simulink model "dds_cwg_32k_nb_half"  (R2018a)
settings: Solver=VariableStepDiscrete  StartTime=0.0  StopTime=(2^16)*20  RelTol=1e-3
undefined symbols (not defined in the file or in its folder): fft_stages, pfb_coeff_gen_calc
libraries: xbsIndex_r4 x11238, casper_library_misc x13, casper_library_delays x2, xps_library x1
(part 14 of 69)

== system dds_cwg_32k_nb_half/DDC/dec_fir_async1 ==
  sync_in : Inport
  dv_in : Inport  Port=2
  real1 : Inport  Port=3
  imag1 : Inport  Port=4
  real2 : Inport  Port=5
  imag2 : Inport  Port=6
  real3 : Inport  Port=7
  imag3 : Inport  Port=8
  real4 : Inport  Port=9
  imag4 : Inport  Port=10
  real5 : Inport  Port=11
  imag5 : Inport  Port=12
  real6 : Inport  Port=13
  imag6 : Inport  Port=14
  real7 : Inport  Port=15
  imag7 : Inport  Port=16
  real8 : Inport  Port=17
  imag8 : Inport  Port=18
  real9 : Inport  Port=19
  imag9 : Inport  Port=20
  real10 : Inport  Port=21
  imag10 : Inport  Port=22
  real11 : Inport  Port=23
  imag11 : Inport  Port=24
  real12 : Inport  Port=25
  imag12 : Inport  Port=26
  real13 : Inport  Port=27
  imag13 : Inport  Port=28
  real14 : Inport  Port=29
  imag14 : Inport  Port=30
  real15 : Inport  Port=31
  imag15 : Inport  Port=32
  real16 : Inport  Port=33
  imag16 : Inport  Port=34
  real17 : Inport  Port=35
  imag17 : Inport  Port=36
  real18 : Inport  Port=37
  imag18 : Inport  Port=38
  real19 : Inport  Port=39
  imag19 : Inport  Port=40
  real20 : Inport  Port=41
  imag20 : Inport  Port=42
  real21 : Inport  Port=43
  imag21 : Inport  Port=44
  real22 : Inport  Port=45
  imag22 : Inport  Port=46
  real23 : Inport  Port=47
  imag23 : Inport  Port=48
  real24 : Inport  Port=49
  imag24 : Inport  Port=50
  real25 : Inport  Port=51
  imag25 : Inport  Port=52
  real26 : Inport  Port=53
  imag26 : Inport  Port=54
  real27 : Inport  Port=55
  imag27 : Inport  Port=56
  real28 : Inport  Port=57
  imag28 : Inport  Port=58
  real29 : Inport  Port=59
  imag29 : Inport  Port=60
  real30 : Inport  Port=61
  imag30 : Inport  Port=62
  real31 : Inport  Port=63
  imag31 : Inport  Port=64
  real32 : Inport  Port=65
  imag32 : Inport  Port=66
  convert1 : xbsIndex_r4/Convert  gui_display_data_type=Fixed-point  arith_type="Signed  (2's comp)"  n_bits=18  bin_pt=17  float_type=Single  exp_bits=8  fraction_bits=24  quantization="Round  (unbiased: +/- Inf)"  overflow=Wrap  en=off  latency=7  pipeline=off  dbl_ovrd=off  block_type=convert
  convert2 : xbsIndex_r4/Convert  gui_display_data_type=Fixed-point  arith_type="Signed  (2's comp)"  n_bits=18  bin_pt=17  float_type=Single  exp_bits=8  fraction_bits=24  quantization="Round  (unbiased: +/- Inf)"  overflow=Wrap  en=off  latency=7  pipeline=off  dbl_ovrd=off  block_type=convert
  dv_delay : xbsIndex_r4/Delay  rst=off  infoeditControl=Selection of Reset will increase slice count due to use of real FFs and instead of SRLs  en=off  latency=2  reg_retiming=off  dbl_ovrd=off  block_type=delay
  fir_col_async1 : Subsystem  AncestorBlock=casper_library_downconverter/fir_col_async  mask(fir_col_async){n_inputs=32, coeff=[-0.001506    -0.00204   -0.002487    -0.00285   -0.003135   -0.003345   -0.003487   -0.003566   -0.003589   -0.003562   -0.003491   -0.003383   -0.003243   -0.003077   -0.002892   -0.002692   -0.002483   -0.002269   -0.002054   -0.001841   -0.001634   -0.001436   -0.001247   -0.001071   -0.000909    -0.00076   -0.000626   -0.000507   -0.000402   -0.000312   -0.000234   -0.000339], add_latency=7, mult_latency=7, coeff_bit_width=18, coeff_bin_pt=17, first_stage_hdl=on, adder_imp=DSP48, async=on, bus_input=off, input_width=0, input_bp=0, input_type=Signed, dbl=on}
      mask prompts: n_inputs "Inputs"; coeff "Coefficients"; add_latency "Add latency"; mult_latency "Mult Latency"; coeff_bit_width "Coefficient bit width"; coeff_bin_pt "Coefficient binary point"; first_stage_hdl "Implement first stage of adder trees on output as behavioural HDL"; adder_imp "Adder implementation"; async "Asynchronous ops"; bus_input "Bus input"; input_width "Input bitwidth"; input_bp "Input binary point"; input_type "Input datatype"; dbl "Double col"
      mask init:
      | fir_col_async_init(gcb);
      mask Help: eval('xlWeb(''http://casper.berkeley.edu/wiki/Fir_col'')')
      mask TypeOptions adder_imp: Behavioral | Fabric | DSP48
      mask Callback bus_input:
      | onoff = get_param(gcb, 'bus_input');
      | set_param_state(gcb, 'input_width', onoff)
      | set_param_state(gcb, 'input_bp', onoff)
      | set_param_state(gcb, 'input_type', onoff)
      mask TypeOptions input_type: Signed | Unsigned
  fir_col_async2 : Subsystem  AncestorBlock=casper_library_downconverter/fir_col_async  mask(fir_col_async){n_inputs=32, coeff=[0.035749    0.035589    0.035272    0.034799    0.034177     0.03341    0.032507    0.031476    0.030327    0.029072     0.02772    0.026286    0.024783    0.023223     0.02162    0.019988    0.018341    0.016693    0.015055     0.01344     0.01186    0.010325    0.008847    0.007432    0.006089    0.004826    0.003646    0.002555    0.001555    0.000649   -0.000163   -0.000881], add_latency=7, mult_latency=7, coeff_bit_width=18, coeff_bin_pt=17, first_stage_hdl=on, adder_imp=DSP48, async=on, bus_input=off, input_width=0, input_bp=0, input_type=Signed, dbl=on}
      mask prompts: n_inputs "Inputs"; coeff "Coefficients"; add_latency "Add latency"; mult_latency "Mult Latency"; coeff_bit_width "Coefficient bit width"; coeff_bin_pt "Coefficient binary point"; first_stage_hdl "Implement first stage of adder trees on output as behavioural HDL"; adder_imp "Adder implementation"; async "Asynchronous ops"; bus_input "Bus input"; input_width "Input bitwidth"; input_bp "Input binary point"; input_type "Input datatype"; dbl "Double col"
      mask init:
      | fir_col_async_init(gcb);
      mask Help: eval('xlWeb(''http://casper.berkeley.edu/wiki/Fir_col'')')
      mask TypeOptions adder_imp: Behavioral | Fabric | DSP48
      mask Callback bus_input:
      | onoff = get_param(gcb, 'bus_input');
      | set_param_state(gcb, 'input_width', onoff)
      | set_param_state(gcb, 'input_bp', onoff)
      | set_param_state(gcb, 'input_type', onoff)
      mask TypeOptions input_type: Signed | Unsigned
  imag_sum : Subsystem  AncestorBlock=casper_library_misc/adder_tree  mask(adder_tree){n_inputs=2, csp_latency=7, adder_imp=DSP48, first_stage_hdl=off, floating_point=off, dvalid_en=on, float_type=single, frac_width=0, exp_width=0}
      mask prompts: n_inputs "Number of Inputs"; csp_latency "Add Latency"; adder_imp "Adder implementation"; first_stage_hdl "Use behavioural HDL for first stage of adders"; floating_point "floating point"; float_type "float type"; frac_width "fraction length"; exp_width "exponent length"
      mask help:
      | Sums all inputs using a tree of adds and delays.
      |
      | Number of inputs: The number of inputs to the block to be summed
      | Add latency: The number of clock cycles to perform one addition (affects timing)..
      | Adder implementation: choice of fabric or DSP48E core, or behavioral HDL
      | Use behavioural HDL for first stage of adders: Causes the first stage of adders to be absorbed into DSP blocks if multipliers precede them (Virtex 5). Overrides Adder implementation
      mask init:
      | adder_tree_init(gcb, ...
      |     'n_inputs', n_inputs, ...
      |     'csp_latency', csp_latency, ...
      |     'adder_imp', adder_imp, ...
      |     'dvalid_en', dvalid_en, ...
      |     'floating_point', floating_point, ...
      |     'float_type', float_type, ...
      |     'exp_width', exp_width, ...
      |     'frac_width', frac_width, ...     
      |     'first_stage_hdl', first_stage_hdl);
      settings: AttributesFormatString=latency 7
      mask Help: eval('xlWeb(''http://casper.berkeley.edu/wiki/Adder_tree'')')
      mask TypeOptions adder_imp: Behavioral | Fabric | DSP48
      mask Callback floating_point:
      | onoff = get_param(gcb, 'floating_point');
      | if strcmp(onoff,'on')
      |     enable_fixpt = 'off'
      |     set_param_state(gcb, 'float_type', 'on')
      | 
      |     f_type = get_param(gcb, 'float_type')
      |     if strcmp(f_type,'custom')
      |         set_param_state(gcb, 'exp_width', 'on')
      |         set_param_state(gcb, 'frac_width', 'on')
      |     else
      |         set_param_state(gcb, 'exp_width', 'off')
      |         set_param_state(gcb, 'frac_width', 'off')
      |     end
      | 
      | 
      | else
      |     enable_fixpt = 'on'
      |     set_param_state(gcb, 'float_type', 'off')
      |     set_param_state(gcb, 'exp_width', 'off')
      |     set_param_state(gcb, 'frac_width', 'off')
      | end
      mask TypeOptions float_type: single | custom
      mask Callback float_type:
      | f_type = get_param(gcb, 'float_type')
      | if strcmp(f_type,'custom')
      |     set_param_state(gcb, 'exp_width', 'on')
      |     set_param_state(gcb, 'frac_width', 'on')
      | else
      |     set_param_state(gcb, 'exp_width', 'off')
      |     set_param_state(gcb, 'frac_width', 'off')
      | end
  real_sum : Subsystem  AncestorBlock=casper_library_misc/adder_tree  mask(adder_tree){n_inputs=2, csp_latency=7, adder_imp=DSP48, first_stage_hdl=off, floating_point=off, dvalid_en=on, float_type=single, frac_width=0, exp_width=0}
      mask prompts: n_inputs "Number of Inputs"; csp_latency "Add Latency"; adder_imp "Adder implementation"; first_stage_hdl "Use behavioural HDL for first stage of adders"; floating_point "floating point"; float_type "float type"; frac_width "fraction length"; exp_width "exponent length"
      mask help:
      | Sums all inputs using a tree of adds and delays.
      |
      | Number of inputs: The number of inputs to the block to be summed
      | Add latency: The number of clock cycles to perform one addition (affects timing)..
      | Adder implementation: choice of fabric or DSP48E core, or behavioral HDL
      | Use behavioural HDL for first stage of adders: Causes the first stage of adders to be absorbed into DSP blocks if multipliers precede them (Virtex 5). Overrides Adder implementation
      mask init: same as dds_cwg_32k_nb_half/DDC/dec_fir_async1/imag_sum
      settings: AttributesFormatString=latency 7
      mask Help: eval('xlWeb(''http://casper.berkeley.edu/wiki/Adder_tree'')')
      mask TypeOptions adder_imp: Behavioral | Fabric | DSP48
      mask Callback floating_point:
      | onoff = get_param(gcb, 'floating_point');
      | if strcmp(onoff,'on')
      |     enable_fixpt = 'off'
      |     set_param_state(gcb, 'float_type', 'on')
      | 
      |     f_type = get_param(gcb, 'float_type')
      |     if strcmp(f_type,'custom')
      |         set_param_state(gcb, 'exp_width', 'on')
      |         set_param_state(gcb, 'frac_width', 'on')
      |     else
      |         set_param_state(gcb, 'exp_width', 'off')
      |         set_param_state(gcb, 'frac_width', 'off')
      |     end
      | 
      | 
      | else
      |     enable_fixpt = 'on'
      |     set_param_state(gcb, 'float_type', 'off')
      |     set_param_state(gcb, 'exp_width', 'off')
      |     set_param_state(gcb, 'frac_width', 'off')
      | end
      mask TypeOptions float_type: single | custom
      mask Callback float_type:
      | f_type = get_param(gcb, 'float_type')
      | if strcmp(f_type,'custom')
      |     set_param_state(gcb, 'exp_width', 'on')
      |     set_param_state(gcb, 'frac_width', 'on')
      | else
      |     set_param_state(gcb, 'exp_width', 'off')
      |     set_param_state(gcb, 'frac_width', 'off')
      | end
  ri_to_c : casper_library_misc/ri_to_c
      settings: SourceProductName=CASPER DSP Blockset
  shift1 : xbsIndex_r4/Shift  shift_dir=Left  shift_bits=1  en=off  latency=1  precision=Full  arith_type="Signed  (2's comp)"  n_bits=16  bin_pt=14  quantization=Truncate  overflow=Wrap  dbl_ovrd=off  block_type=shift
  shift2 : xbsIndex_r4/Shift  shift_dir=Left  shift_bits=1  en=off  latency=1  precision=Full  arith_type="Signed  (2's comp)"  n_bits=16  bin_pt=14  quantization=Truncate  overflow=Wrap  dbl_ovrd=off  block_type=shift
  sync_delay : xbsIndex_r4/Delay  rst=off  infoeditControl=Selection of Reset will increase slice count due to use of real FFs and instead of SRLs  en=on  latency=56  reg_retiming=off  dbl_ovrd=off  block_type=delay
  sync_out : Outport
  dout : Outport  Port=2
  dv_out : Outport  Port=3
  wires:
  sync_in/1 -> sync_delay/1
  dv_in/1 -> dv_delay/1, sync_delay/2, fir_col_async1/129(dv), fir_col_async2/129(dv), real_sum/1(dv_in), imag_sum/1(dv_in)
  dv_delay/1 -> dv_out/1
  real1/1 -> fir_col_async1/1(real1)
  imag1/1 -> fir_col_async1/2(imag1)
  real2/1 -> fir_col_async1/3(real2)
  imag2/1 -> fir_col_async1/4(imag2)
  real3/1 -> fir_col_async1/5(real3)
  imag3/1 -> fir_col_async1/6(imag3)
  real4/1 -> fir_col_async1/7(real4)
  imag4/1 -> fir_col_async1/8(imag4)
  real5/1 -> fir_col_async1/9(real5)
  imag5/1 -> fir_col_async1/10(imag5)
  real6/1 -> fir_col_async1/11(real6)
  imag6/1 -> fir_col_async1/12(imag6)
  real7/1 -> fir_col_async1/13(real7)
  imag7/1 -> fir_col_async1/14(imag7)
  real8/1 -> fir_col_async1/15(real8)
  imag8/1 -> fir_col_async1/16(imag8)
  real9/1 -> fir_col_async1/17(real9)
  imag9/1 -> fir_col_async1/18(imag9)
  real10/1 -> fir_col_async1/19(real10)
  imag10/1 -> fir_col_async1/20(imag10)
  real11/1 -> fir_col_async1/21(real11)
  imag11/1 -> fir_col_async1/22(imag11)
  real12/1 -> fir_col_async1/23(real12)
  imag12/1 -> fir_col_async1/24(imag12)
  real13/1 -> fir_col_async1/25(real13)
  imag13/1 -> fir_col_async1/26(imag13)
  real14/1 -> fir_col_async1/27(real14)
  imag14/1 -> fir_col_async1/28(imag14)
  real15/1 -> fir_col_async1/29(real15)
  imag15/1 -> fir_col_async1/30(imag15)
  real16/1 -> fir_col_async1/31(real16)
  imag16/1 -> fir_col_async1/32(imag16)
  real17/1 -> fir_col_async1/33(real17)
  imag17/1 -> fir_col_async1/34(imag17)
  real18/1 -> fir_col_async1/35(real18)
  imag18/1 -> fir_col_async1/36(imag18)
  real19/1 -> fir_col_async1/37(real19)
  imag19/1 -> fir_col_async1/38(imag19)
  real20/1 -> fir_col_async1/39(real20)
  imag20/1 -> fir_col_async1/40(imag20)
  real21/1 -> fir_col_async1/41(real21)
  imag21/1 -> fir_col_async1/42(imag21)
  real22/1 -> fir_col_async1/43(real22)
  imag22/1 -> fir_col_async1/44(imag22)
  real23/1 -> fir_col_async1/45(real23)
  imag23/1 -> fir_col_async1/46(imag23)
  real24/1 -> fir_col_async1/47(real24)
  imag24/1 -> fir_col_async1/48(imag24)
  real25/1 -> fir_col_async1/49(real25)
  imag25/1 -> fir_col_async1/50(imag25)
  real26/1 -> fir_col_async1/51(real26)
  imag26/1 -> fir_col_async1/52(imag26)
  real27/1 -> fir_col_async1/53(real27)
  imag27/1 -> fir_col_async1/54(imag27)
  real28/1 -> fir_col_async1/55(real28)
  imag28/1 -> fir_col_async1/56(imag28)
  real29/1 -> fir_col_async1/57(real29)
  imag29/1 -> fir_col_async1/58(imag29)
  real30/1 -> fir_col_async1/59(real30)
  imag30/1 -> fir_col_async1/60(imag30)
  real31/1 -> fir_col_async1/61(real31)
  imag31/1 -> fir_col_async1/62(imag31)
  real32/1 -> fir_col_async1/63(real32)
  imag32/1 -> fir_col_async1/64(imag32)
  fir_col_async1/129(real_sum) -> real_sum/3(din1)
  fir_col_async1/130(imag_sum) -> imag_sum/3(din1)
  fir_col_async1/1(real_out1) -> fir_col_async2/1(real1)
  fir_col_async1/2(imag_out1) -> fir_col_async2/2(imag1)
  fir_col_async1/3(real_out2) -> fir_col_async2/3(real2)
  fir_col_async1/4(imag_out2) -> fir_col_async2/4(imag2)
  fir_col_async1/5(real_out3) -> fir_col_async2/5(real3)
  fir_col_async1/6(imag_out3) -> fir_col_async2/6(imag3)
  fir_col_async1/7(real_out4) -> fir_col_async2/7(real4)
  fir_col_async1/8(imag_out4) -> fir_col_async2/8(imag4)
  fir_col_async1/9(real_out5) -> fir_col_async2/9(real5)
  fir_col_async1/10(imag_out5) -> fir_col_async2/10(imag5)
  fir_col_async1/11(real_out6) -> fir_col_async2/11(real6)
  fir_col_async1/12(imag_out6) -> fir_col_async2/12(imag6)
  fir_col_async1/13(real_out7) -> fir_col_async2/13(real7)
  fir_col_async1/14(imag_out7) -> fir_col_async2/14(imag7)
  fir_col_async1/15(real_out8) -> fir_col_async2/15(real8)
  fir_col_async1/16(imag_out8) -> fir_col_async2/16(imag8)
  fir_col_async1/17(real_out9) -> fir_col_async2/17(real9)
  fir_col_async1/18(imag_out9) -> fir_col_async2/18(imag9)
  fir_col_async1/19(real_out10) -> fir_col_async2/19(real10)
  fir_col_async1/20(imag_out10) -> fir_col_async2/20(imag10)
  fir_col_async1/21(real_out11) -> fir_col_async2/21(real11)
  fir_col_async1/22(imag_out11) -> fir_col_async2/22(imag11)
  fir_col_async1/23(real_out12) -> fir_col_async2/23(real12)
  fir_col_async1/24(imag_out12) -> fir_col_async2/24(imag12)
  fir_col_async1/25(real_out13) -> fir_col_async2/25(real13)
  fir_col_async1/26(imag_out13) -> fir_col_async2/26(imag13)
  fir_col_async1/27(real_out14) -> fir_col_async2/27(real14)
  fir_col_async1/28(imag_out14) -> fir_col_async2/28(imag14)
  fir_col_async1/29(real_out15) -> fir_col_async2/29(real15)
  fir_col_async1/30(imag_out15) -> fir_col_async2/30(imag15)
  fir_col_async1/31(real_out16) -> fir_col_async2/31(real16)
  fir_col_async1/32(imag_out16) -> fir_col_async2/32(imag16)
  fir_col_async1/33(real_out17) -> fir_col_async2/33(real17)
  fir_col_async1/34(imag_out17) -> fir_col_async2/34(imag17)
  fir_col_async1/35(real_out18) -> fir_col_async2/35(real18)
  fir_col_async1/36(imag_out18) -> fir_col_async2/36(imag18)
  fir_col_async1/37(real_out19) -> fir_col_async2/37(real19)
  fir_col_async1/38(imag_out19) -> fir_col_async2/38(imag19)
  fir_col_async1/39(real_out20) -> fir_col_async2/39(real20)
  fir_col_async1/40(imag_out20) -> fir_col_async2/40(imag20)
  fir_col_async1/41(real_out21) -> fir_col_async2/41(real21)
  fir_col_async1/42(imag_out21) -> fir_col_async2/42(imag21)
  fir_col_async1/43(real_out22) -> fir_col_async2/43(real22)
  fir_col_async1/44(imag_out22) -> fir_col_async2/44(imag22)
  fir_col_async1/45(real_out23) -> fir_col_async2/45(real23)
  fir_col_async1/46(imag_out23) -> fir_col_async2/46(imag23)
  fir_col_async1/47(real_out24) -> fir_col_async2/47(real24)
  fir_col_async1/48(imag_out24) -> fir_col_async2/48(imag24)
  fir_col_async1/49(real_out25) -> fir_col_async2/49(real25)
  fir_col_async1/50(imag_out25) -> fir_col_async2/50(imag25)
  fir_col_async1/51(real_out26) -> fir_col_async2/51(real26)
  fir_col_async1/52(imag_out26) -> fir_col_async2/52(imag26)
  fir_col_async1/53(real_out27) -> fir_col_async2/53(real27)
  fir_col_async1/54(imag_out27) -> fir_col_async2/54(imag27)
  fir_col_async1/55(real_out28) -> fir_col_async2/55(real28)
  fir_col_async1/56(imag_out28) -> fir_col_async2/56(imag28)
  fir_col_async1/57(real_out29) -> fir_col_async2/57(real29)
  fir_col_async1/58(imag_out29) -> fir_col_async2/58(imag29)
  fir_col_async1/59(real_out30) -> fir_col_async2/59(real30)
  fir_col_async1/60(imag_out30) -> fir_col_async2/60(imag30)
  fir_col_async1/61(real_out31) -> fir_col_async2/61(real31)
  fir_col_async1/62(imag_out31) -> fir_col_async2/62(imag31)
  fir_col_async1/63(real_out32) -> fir_col_async2/63(real32)
  fir_col_async1/64(imag_out32) -> fir_col_async2/64(imag32)
  fir_col_async2/129(real_sum) -> real_sum/4(din2)
  fir_col_async2/130(imag_sum) -> imag_sum/4(din2)
  real_sum/2(dout) -> shift1/1
  imag_sum/2(dout) -> shift2/1
  shift1/1 -> convert1/1
  shift2/1 -> convert2/1
  convert1/1 -> ri_to_c/1
  convert2/1 -> ri_to_c/2
  ri_to_c/1 -> dout/1
  real_sum/1(sync_out) -> sync_out/1
  sync_delay/1 -> real_sum/2(sync), imag_sum/2(sync)
  fir_col_async2/65(real_back_out1) -> fir_col_async1/65(real_back1)
  fir_col_async2/66(imag_back_out1) -> fir_col_async1/66(imag_back1)
  fir_col_async2/67(real_back_out2) -> fir_col_async1/67(real_back2)
  fir_col_async2/68(imag_back_out2) -> fir_col_async1/68(imag_back2)
  fir_col_async2/69(real_back_out3) -> fir_col_async1/69(real_back3)
  fir_col_async2/70(imag_back_out3) -> fir_col_async1/70(imag_back3)
  fir_col_async2/71(real_back_out4) -> fir_col_async1/71(real_back4)
  fir_col_async2/72(imag_back_out4) -> fir_col_async1/72(imag_back4)
  fir_col_async2/73(real_back_out5) -> fir_col_async1/73(real_back5)
  fir_col_async2/74(imag_back_out5) -> fir_col_async1/74(imag_back5)
  fir_col_async2/75(real_back_out6) -> fir_col_async1/75(real_back6)
  fir_col_async2/76(imag_back_out6) -> fir_col_async1/76(imag_back6)
  fir_col_async2/77(real_back_out7) -> fir_col_async1/77(real_back7)
  fir_col_async2/78(imag_back_out7) -> fir_col_async1/78(imag_back7)
  fir_col_async2/79(real_back_out8) -> fir_col_async1/79(real_back8)
  fir_col_async2/80(imag_back_out8) -> fir_col_async1/80(imag_back8)
  fir_col_async2/81(real_back_out9) -> fir_col_async1/81(real_back9)
  fir_col_async2/82(imag_back_out9) -> fir_col_async1/82(imag_back9)
  fir_col_async2/83(real_back_out10) -> fir_col_async1/83(real_back10)
  fir_col_async2/84(imag_back_out10) -> fir_col_async1/84(imag_back10)
  fir_col_async2/85(real_back_out11) -> fir_col_async1/85(real_back11)
  fir_col_async2/86(imag_back_out11) -> fir_col_async1/86(imag_back11)
  fir_col_async2/87(real_back_out12) -> fir_col_async1/87(real_back12)
  fir_col_async2/88(imag_back_out12) -> fir_col_async1/88(imag_back12)
  fir_col_async2/89(real_back_out13) -> fir_col_async1/89(real_back13)
  fir_col_async2/90(imag_back_out13) -> fir_col_async1/90(imag_back13)
  fir_col_async2/91(real_back_out14) -> fir_col_async1/91(real_back14)
  fir_col_async2/92(imag_back_out14) -> fir_col_async1/92(imag_back14)
  fir_col_async2/93(real_back_out15) -> fir_col_async1/93(real_back15)
  fir_col_async2/94(imag_back_out15) -> fir_col_async1/94(imag_back15)
  fir_col_async2/95(real_back_out16) -> fir_col_async1/95(real_back16)
  fir_col_async2/96(imag_back_out16) -> fir_col_async1/96(imag_back16)
  fir_col_async2/97(real_back_out17) -> fir_col_async1/97(real_back17)
  fir_col_async2/98(imag_back_out17) -> fir_col_async1/98(imag_back17)
  fir_col_async2/99(real_back_out18) -> fir_col_async1/99(real_back18)
  fir_col_async2/100(imag_back_out18) -> fir_col_async1/100(imag_back18)
  fir_col_async2/101(real_back_out19) -> fir_col_async1/101(real_back19)
  fir_col_async2/102(imag_back_out19) -> fir_col_async1/102(imag_back19)
  fir_col_async2/103(real_back_out20) -> fir_col_async1/103(real_back20)
  fir_col_async2/104(imag_back_out20) -> fir_col_async1/104(imag_back20)
  fir_col_async2/105(real_back_out21) -> fir_col_async1/105(real_back21)
  fir_col_async2/106(imag_back_out21) -> fir_col_async1/106(imag_back21)
  fir_col_async2/107(real_back_out22) -> fir_col_async1/107(real_back22)
  fir_col_async2/108(imag_back_out22) -> fir_col_async1/108(imag_back22)
  fir_col_async2/109(real_back_out23) -> fir_col_async1/109(real_back23)
  fir_col_async2/110(imag_back_out23) -> fir_col_async1/110(imag_back23)
  fir_col_async2/111(real_back_out24) -> fir_col_async1/111(real_back24)
  fir_col_async2/112(imag_back_out24) -> fir_col_async1/112(imag_back24)
  fir_col_async2/113(real_back_out25) -> fir_col_async1/113(real_back25)
  fir_col_async2/114(imag_back_out25) -> fir_col_async1/114(imag_back25)
  fir_col_async2/115(real_back_out26) -> fir_col_async1/115(real_back26)
  fir_col_async2/116(imag_back_out26) -> fir_col_async1/116(imag_back26)
  fir_col_async2/117(real_back_out27) -> fir_col_async1/117(real_back27)
  fir_col_async2/118(imag_back_out27) -> fir_col_async1/118(imag_back27)
  fir_col_async2/119(real_back_out28) -> fir_col_async1/119(real_back28)
  fir_col_async2/120(imag_back_out28) -> fir_col_async1/120(imag_back28)
  fir_col_async2/121(real_back_out29) -> fir_col_async1/121(real_back29)
  fir_col_async2/122(imag_back_out29) -> fir_col_async1/122(imag_back29)
  fir_col_async2/123(real_back_out30) -> fir_col_async1/123(real_back30)
  fir_col_async2/124(imag_back_out30) -> fir_col_async1/124(imag_back30)
  fir_col_async2/125(real_back_out31) -> fir_col_async1/125(real_back31)
  fir_col_async2/126(imag_back_out31) -> fir_col_async1/126(imag_back31)
  fir_col_async2/127(real_back_out32) -> fir_col_async1/127(real_back32)
  fir_col_async2/128(imag_back_out32) -> fir_col_async1/128(imag_back32)
  fir_col_async2/1(real_out1) -> fir_col_async2/65(real_back1)
  fir_col_async2/2(imag_out1) -> fir_col_async2/66(imag_back1)
  fir_col_async2/3(real_out2) -> fir_col_async2/67(real_back2)
  fir_col_async2/4(imag_out2) -> fir_col_async2/68(imag_back2)
  fir_col_async2/5(real_out3) -> fir_col_async2/69(real_back3)
  fir_col_async2/6(imag_out3) -> fir_col_async2/70(imag_back3)
  fir_col_async2/7(real_out4) -> fir_col_async2/71(real_back4)
  fir_col_async2/8(imag_out4) -> fir_col_async2/72(imag_back4)
  fir_col_async2/9(real_out5) -> fir_col_async2/73(real_back5)
  fir_col_async2/10(imag_out5) -> fir_col_async2/74(imag_back5)
  fir_col_async2/11(real_out6) -> fir_col_async2/75(real_back6)
  fir_col_async2/12(imag_out6) -> fir_col_async2/76(imag_back6)
  fir_col_async2/13(real_out7) -> fir_col_async2/77(real_back7)
  fir_col_async2/14(imag_out7) -> fir_col_async2/78(imag_back7)
  fir_col_async2/15(real_out8) -> fir_col_async2/79(real_back8)
  fir_col_async2/16(imag_out8) -> fir_col_async2/80(imag_back8)
  fir_col_async2/17(real_out9) -> fir_col_async2/81(real_back9)
  fir_col_async2/18(imag_out9) -> fir_col_async2/82(imag_back9)
  fir_col_async2/19(real_out10) -> fir_col_async2/83(real_back10)
  fir_col_async2/20(imag_out10) -> fir_col_async2/84(imag_back10)
  fir_col_async2/21(real_out11) -> fir_col_async2/85(real_back11)
  fir_col_async2/22(imag_out11) -> fir_col_async2/86(imag_back11)
  fir_col_async2/23(real_out12) -> fir_col_async2/87(real_back12)
  fir_col_async2/24(imag_out12) -> fir_col_async2/88(imag_back12)
  fir_col_async2/25(real_out13) -> fir_col_async2/89(real_back13)
  fir_col_async2/26(imag_out13) -> fir_col_async2/90(imag_back13)
  fir_col_async2/27(real_out14) -> fir_col_async2/91(real_back14)
  fir_col_async2/28(imag_out14) -> fir_col_async2/92(imag_back14)
  fir_col_async2/29(real_out15) -> fir_col_async2/93(real_back15)
  fir_col_async2/30(imag_out15) -> fir_col_async2/94(imag_back15)
  fir_col_async2/31(real_out16) -> fir_col_async2/95(real_back16)
  fir_col_async2/32(imag_out16) -> fir_col_async2/96(imag_back16)
  fir_col_async2/33(real_out17) -> fir_col_async2/97(real_back17)
  fir_col_async2/34(imag_out17) -> fir_col_async2/98(imag_back17)
  fir_col_async2/35(real_out18) -> fir_col_async2/99(real_back18)
  fir_col_async2/36(imag_out18) -> fir_col_async2/100(imag_back18)
  fir_col_async2/37(real_out19) -> fir_col_async2/101(real_back19)
  fir_col_async2/38(imag_out19) -> fir_col_async2/102(imag_back19)
  fir_col_async2/39(real_out20) -> fir_col_async2/103(real_back20)
  fir_col_async2/40(imag_out20) -> fir_col_async2/104(imag_back20)
  fir_col_async2/41(real_out21) -> fir_col_async2/105(real_back21)
  fir_col_async2/42(imag_out21) -> fir_col_async2/106(imag_back21)
  fir_col_async2/43(real_out22) -> fir_col_async2/107(real_back22)
  fir_col_async2/44(imag_out22) -> fir_col_async2/108(imag_back22)
  fir_col_async2/45(real_out23) -> fir_col_async2/109(real_back23)
  fir_col_async2/46(imag_out23) -> fir_col_async2/110(imag_back23)
  fir_col_async2/47(real_out24) -> fir_col_async2/111(real_back24)
  fir_col_async2/48(imag_out24) -> fir_col_async2/112(imag_back24)
  fir_col_async2/49(real_out25) -> fir_col_async2/113(real_back25)
  fir_col_async2/50(imag_out25) -> fir_col_async2/114(imag_back25)
  fir_col_async2/51(real_out26) -> fir_col_async2/115(real_back26)
  fir_col_async2/52(imag_out26) -> fir_col_async2/116(imag_back26)
  fir_col_async2/53(real_out27) -> fir_col_async2/117(real_back27)
  fir_col_async2/54(imag_out27) -> fir_col_async2/118(imag_back27)
  fir_col_async2/55(real_out28) -> fir_col_async2/119(real_back28)
  fir_col_async2/56(imag_out28) -> fir_col_async2/120(imag_back28)
  fir_col_async2/57(real_out29) -> fir_col_async2/121(real_back29)
  fir_col_async2/58(imag_out29) -> fir_col_async2/122(imag_back29)
  fir_col_async2/59(real_out30) -> fir_col_async2/123(real_back30)
  fir_col_async2/60(imag_out30) -> fir_col_async2/124(imag_back30)
  fir_col_async2/61(real_out31) -> fir_col_async2/125(real_back31)
  fir_col_async2/62(imag_out31) -> fir_col_async2/126(imag_back31)
  fir_col_async2/63(real_out32) -> fir_col_async2/127(real_back32)
  fir_col_async2/64(imag_out32) -> fir_col_async2/128(imag_back32)
